simulink model "analise_discreto"  (R2025a)
settings: Solver=VariableStepAuto  StartTime=0.0  StopTime=150  RelTol=1e-3
values from neighbouring files (symbols this model uses):
  alpha = 0.1    [simulink_constants.m]
  Delay = 0.1    [simulink_constants.m]
  Ubar = 5    [simulink_constants.m]
  Ybar = 3.47    [simulink_constants.m]
undefined symbols (not defined in the file or in its folder): beta, dspblkCoreblockFVToolHelper, gamma, gcbh, kpd_disc, kpp_disc
libraries: simulink x2, cstblocks x1
settings Model: Creator=joaof  LastModifiedBy=joaof

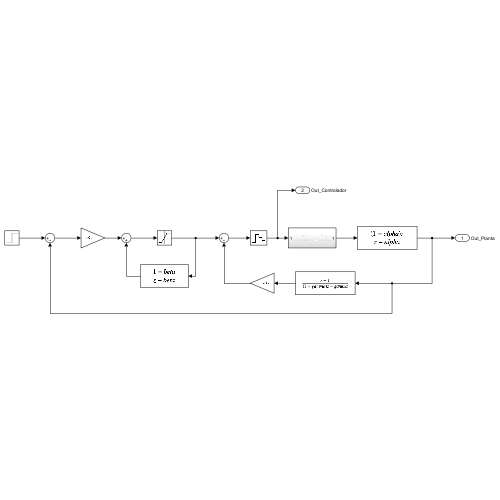
[thumbnail: Simulink's stored preview of the top-level diagram]
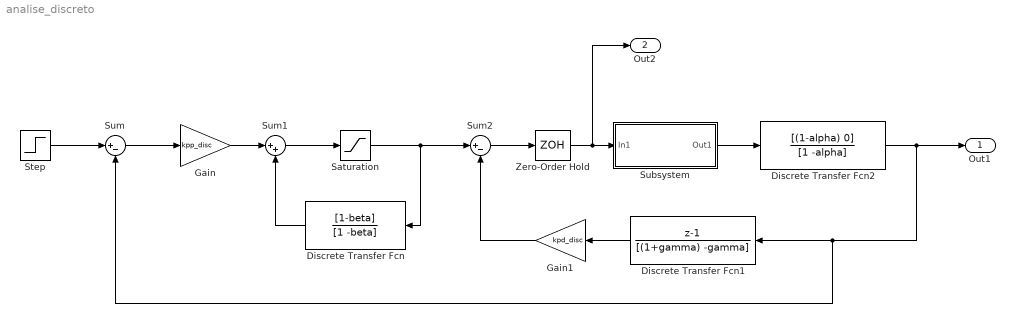
== system analise_discreto ==
  Discrete Transfer Fcn : DiscreteTransferFcn  LoadFcn=dspblkCoreblockFVToolHelper(gcbh,'load');  Numerator=[1-beta]  Denominator=[1 -beta]
      settings: CopyFcn=dspblkCoreblockFVToolHelper(gcbh,'copy');  DeleteFcn=dspblkCoreblockFVToolHelper(gcbh,'close');  ModelCloseFcn=dspblkCoreblockFVToolHelper(gcbh,'close');  PreSaveFcn=dspblkCoreblockFVToolHelper(gcbh,'presave');  PostSaveFcn=dspblkCoreblockFVToolHelper(gcbh,'postsave');  CloseFcn=dspblkCoreblockFVToolHelper(gcbh,'close');
  Discrete Transfer Fcn1 : DiscreteTransferFcn  LoadFcn=dspblkCoreblockFVToolHelper(gcbh,'load');  Numerator=[1 -1]  Denominator=[(1+gamma) -gamma]
      settings: CopyFcn=dspblkCoreblockFVToolHelper(gcbh,'copy');  DeleteFcn=dspblkCoreblockFVToolHelper(gcbh,'close');  ModelCloseFcn=dspblkCoreblockFVToolHelper(gcbh,'close');  PreSaveFcn=dspblkCoreblockFVToolHelper(gcbh,'presave');  PostSaveFcn=dspblkCoreblockFVToolHelper(gcbh,'postsave');  CloseFcn=dspblkCoreblockFVToolHelper(gcbh,'close');
  Discrete Transfer Fcn2 : DiscreteTransferFcn  LoadFcn=dspblkCoreblockFVToolHelper(gcbh,'load');  Numerator=[(1-alpha) 0]  Denominator=[1 -alpha]
      settings: CopyFcn=dspblkCoreblockFVToolHelper(gcbh,'copy');  DeleteFcn=dspblkCoreblockFVToolHelper(gcbh,'close');  ModelCloseFcn=dspblkCoreblockFVToolHelper(gcbh,'close');  PreSaveFcn=dspblkCoreblockFVToolHelper(gcbh,'presave');  PostSaveFcn=dspblkCoreblockFVToolHelper(gcbh,'postsave');  CloseFcn=dspblkCoreblockFVToolHelper(gcbh,'close');
  Gain : Gain  Gain=kpp_disc
  Gain1 : Gain  Gain=kpd_disc
  Saturation : Saturate  UpperLimit=5  LowerLimit=-5
  Step : Step  SampleTime=0
  Subsystem : Subsystem
  Sum : Sum  Inputs=|+-
  Sum1 : Sum  Inputs=|++
  Sum2 : Sum  Inputs=|+-
  Zero-Order Hold : ZeroOrderHold  SampleTime=-1
  Out1 : Outport  SignalName=Out_Planta
  Out2 : Outport  Port=2  SignalName=Out_Controlador
  wires:
  Gain/1 -> Sum1/1
  Sum1/1 -> Saturation/1
  Saturation/1 -> Sum2/1, Discrete Transfer Fcn/1
  Discrete Transfer Fcn/1 -> Sum1/2
  Sum/1 -> Gain/1
  Step/1 -> Sum/1
  Gain1/1 -> Sum2/2
  Discrete Transfer Fcn1/1 -> Gain1/1
  Sum2/1 -> Zero-Order Hold/1
  Zero-Order Hold/1 -> Subsystem/1(In1), Out2/1
  Discrete Transfer Fcn2/1 -> Sum/2, Discrete Transfer Fcn1/1, Out1/1
  Subsystem/1(Out1) -> Discrete Transfer Fcn2/1

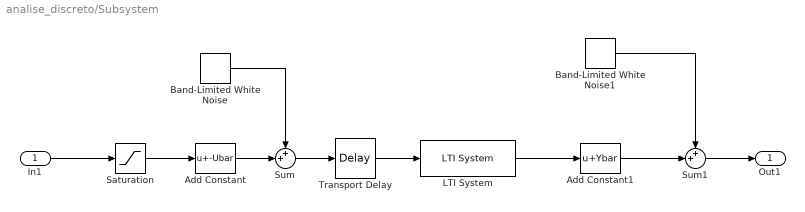
== system analise_discreto/Subsystem ==
  In1 : Inport
  Add Constant : Bias  Bias=-Ubar  SaturateOnIntegerOverflow=off
  Add Constant1 : Bias  Bias=Ybar  SaturateOnIntegerOverflow=off
  Band-Limited White Noise : simulink/Sources/Band-Limited White Noise  Cov=[0.1]  Ts=0.1  seed=[23341]
  Band-Limited White Noise1 : simulink/Sources/Band-Limited White Noise  Cov=[0.1]  Ts=0.1  seed=[23341]
  LTI System : cstblocks/LTI System  sys=G_teste  IC=[]  PadeOrder=0
  Saturation : Saturate  UpperLimit=5  LowerLimit=-5
  Sum : Sum  Inputs=++|
  Sum1 : Sum  Inputs=++|
  Transport Delay : TransportDelay  DelayTime=Delay
  Out1 : Outport
  wires:
  In1/1 -> Saturation/1
  Saturation/1 -> Add Constant/1
  Add Constant/1 -> Sum/2
  Band-Limited White Noise/1 -> Sum/1
  Sum/1 -> Transport Delay/1
  Transport Delay/1 -> LTI System/1
  LTI System/1 -> Add Constant1/1
  Add Constant1/1 -> Sum1/2
  Band-Limited White Noise1/1 -> Sum1/1
  Sum1/1 -> Out1/1
